simulink model "psbdistline"  (Simulink 6.0)
settings: Solver=ode15s  SolverMode=SingleTasking  StartTime=0.0  StopTime=0.1  MaxStep=50e-6  RelTol=1e-3  AbsTol=1e-6
libraries: powerlib2 x10
settings Model: Creator=patrice  LastModifiedBy=batserve  ExtModeTrigMode=oneshot  ExtModeArmWhenConnect=off  ExtModeAutoUpdateStatusClock=off
settings DataIOCC: LimitDataPoints=off  SignalLoggingName=sigsOut
settings OptimizationCC: BooleanDataType=off
settings DebuggingCC: SolverPrmCheckMsg=none
settings HardwareCC: TargetUnknown=on
settings RTWCC: TemplateMakefile=grt_unix.tmf

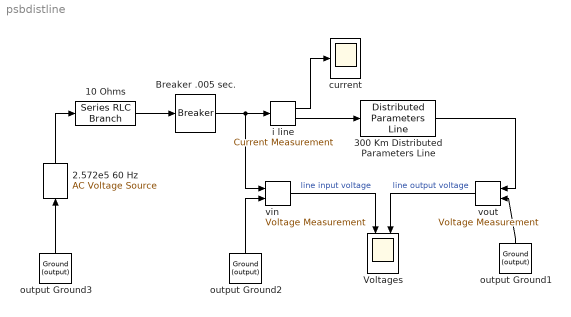
== system psbdistline ==
  10 Ohms : powerlib2/Elements/Series RLC Branch  Tag=PoWeRsYsTeMbLoCk  a=10  b=0  c=inf  mesure=None  PSBOutputType=1
  "2.572e5 60 Hz " : powerlib2/Electrical Sources/AC Voltage Source  Tag=PoWeRsYsTeMbLoCk  Orientation=up  A=(315e3*sqrt(2))/sqrt(30)  P=0  F=60  stime=0  mesure=None  PSBOutputType=1
  300 Km Distributed Parameters Line : powerlib2/Elements/Distributed Parameters Line  Tag=PoWeRsYsTeMbLoCk  n=1  f=60  r=0.2568  l=2.0e-3  c=8.6e-9  lgt=300  x1=[0 -1.992e-09;0.0002737 -2.609e-09;0.0005474 -3.197e-09;0.0008212 -3.752e-09;0.001095 -4.267e-09;0.001369 -4.736e-09]  x2=[0 -1.992e-09;0.0002737 -2.609e-09;0.0005474 -3.197e-09;0.0008212 -3.752e-09;0.001095 -4.267e-09;0.001369 -4.736e-09]  x3=[0 -8.754e-13;0.0002737 -2.116e-12;0.0005474 -3.334e-12;0.0008212 -4.517e-12;0.001095 -5.651e-12;0.001369 -6.726e-12]  x4=[0 -8.754e-13;0.0002737 -2.116e-12;0.0005474 -3.334e-12;0.0008212 -4.517e-12;0.001095 -5.651e-12;0.001369 -6.726e-12]  x5=0.001369  mesure=None  PSBOutputType=111111111111111111111111111111
  Breaker .005 sec. : powerlib2/Elements/Breaker  Tag=PoWeRsYsTeMbLoCk  a=1e-1  c=0  rs=inf  cs=0  times=[ .005 ]  Ts=0  comext=off  mesure=None  PSBOutputType=1
  Voltages : Scope  NumInputPorts=2
      settings: Orientation=down  TickLabels=on  TimeRange=0.1  YMin=-100000~-200000  YMax=100000~200000  DataFormat=Array  MaxDataPoints=5000000
  current : Scope
      settings: TickLabels=on  TimeRange=0.05  YMin=-100000  YMax=100000  DataFormat=Array
  i line : powerlib2/Measurements/Current Measurement  Tag=PoWeRsYsTeMmEaSuReMeNt  PhasorSimulation=off  OutputType=Magnitude  PSBOutputType=01  PSBequivalent=0
  output Ground1 : powerlib2/Connectors/Ground (output)  Tag=PoWeRsYsTeMbLoCk  Orientation=up  PSBOutputType=1
  output Ground2 : powerlib2/Connectors/Ground (output)  Tag=PoWeRsYsTeMbLoCk  Orientation=up  PSBOutputType=1
  output Ground3 : powerlib2/Connectors/Ground (output)  Tag=PoWeRsYsTeMbLoCk  Orientation=up  PSBOutputType=1
  vin : powerlib2/Measurements/Voltage Measurement  Tag=PoWeRsYsTeMmEaSuReMeNt  PhasorSimulation=off  OutputType=Magnitude  PSBOutputType=0  PSBequivalent=0
  vout : powerlib2/Measurements/Voltage Measurement  Tag=PoWeRsYsTeMmEaSuReMeNt  Orientation=left  PhasorSimulation=off  OutputType=Magnitude  PSBOutputType=0  PSBequivalent=0
  wires:
  output Ground2/1 -> vin/2
  Breaker .005 sec./1 -> vin/1, i line/1
  "2.572e5 60 Hz "/1 -> 10 Ohms/1
  10 Ohms/1 -> Breaker .005 sec./1
  output Ground3/1 -> "2.572e5 60 Hz "/1
  i line/2 -> 300 Km Distributed Parameters Line/1
  300 Km Distributed Parameters Line/1 -> vout/1
  output Ground1/1 -> vout/2
  i line/1 -> current/1
  vin/1 -> Voltages/1  "line input voltage"
  vout/1 -> Voltages/2  "line output voltage"
